simulink model "layerInterface"  (Simulink 7.4)
settings: Solver=ode45  StartTime=0.0  StopTime=10.0  RelTol=1e-3
settings Model: Creator=chepeadan  LastModifiedBy=chepeadan

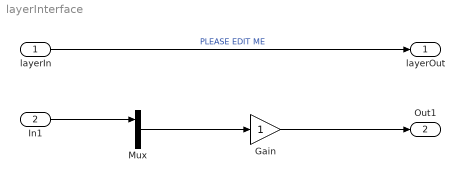
== system layerInterface ==
  layerIn : Inport  OutDataType=fixdt(1, 16)  OutScaling=2^0
  In1 : Inport  Port=2  OutDataType=fixdt(1, 16)  OutScaling=2^0
  Gain : Gain  ParameterDataType=fixdt(1, 16)  ParameterScaling=2^0  OutDataType=fixdt(1, 16)  OutScaling=2^0
  Mux : Mux  Inputs=2
  layerOut : Outport  OutDataType=fixdt(1, 16)  OutScaling=2^0
  Out1 : Outport  Port=2  OutDataType=fixdt(1, 16)  OutScaling=2^0
  wires:
  Mux/1 -> Gain/1
  In1/1 -> Mux/1
  Gain/1 -> Out1/1
  layerIn/1 -> layerOut/1  "PLEASE EDIT ME"
